simulink model "FCS_MPC_6ph_Regelungsmodell"  (R2022a)
settings: Solver=ode23t  StartTime=0.0  StopTime=0.1  RelTol=1e-3  AbsTol=1e-3  EnableMultiTasking=on
values from neighbouring files (symbols this model uses):
  f_c = 100000    [Params_testbench.m]
  L_d = 0.0001473    [Params_testbench.m]
  L_q = 0.0001484    [Params_testbench.m]
  L_x = 0.00005566    (= 5.566e-05)    [Params_testbench.m]
  L_y = L_x    (= 5.566e-05)    [Params_testbench.m]
  p = 5    [Params_testbench.m]
  psi_pm = 0.0048    [Params_testbench.m]
  R_ph = 0.1278    [Params_testbench.m]
  T_100MHz = 1/f_100MHz    (= 1e-08)    [Params_testbench.m]
  u_dc = 36.0    (= 36)    [Params_testbench.m]
libraries: hdlsllib x53, nesl_utility x39, fl_lib x32, ee_lib x12, simulink x8, spsAlphaBetaZerotodq0Lib x1
(part 4 of 8)

== system FCS_MPC_6ph_Regelungsmodell/Microcontroller Software/Phase_voltages_per_switching_state2 ==
  theta_el : Inport
  theta_el_offset_AXI : Inport  Port=2
  u_dc_link_voltage_AXI : Inport  Port=3
  Index : Inport  Port=4
  valid_in_delay_compensation : Inport  Port=5
  valid_in_min_cost_function-and_vopt : Inport  Port=6
  valid_in_ADC : Inport  Port=7
  Add4 : Sum  Inputs=+-  OutDataTypeStr=Inherit: Same as first input
  Add5 : Sum  Inputs=-+  OutDataTypeStr=Inherit: Same as first input
  Add6 : Sum  OutDataTypeStr=Inherit: Same as first input
  Compare Limit_High1 : simulink/Logic and Bit Operations/Compare To Constant  relop=>=  const=2*pi  OutDataTypeStr=boolean
  Compare Limit_Low1 : simulink/Logic and Bit Operations/Compare To Constant  relop=<  const=0  OutDataTypeStr=boolean
  Constant2 : Constant  Value=2*pi  OutDataTypeStr=single  SampleTime=1/100000000
  Constant3 : Constant  Value=2*pi  OutDataTypeStr=single  SampleTime=1/100000000
  Data Type Conversion34 : DataTypeConversion  OutDataTypeStr=single  SaturateOnIntegerOverflow=off  RndMeth=Floor
  Delay{1..11,13..14} (13 alike) : Delay  DelayLength=1
  Detect Rise Positive : hdlsllib/Logic and Bit Operations/Detect Rise Positive  vinit=0  OutDataTypeStr=boolean
      settings: SourceProductBaseCode=SL
  Detect Rise Positive1 : hdlsllib/Logic and Bit Operations/Detect Rise Positive  vinit=0  OutDataTypeStr=boolean
      settings: SourceProductBaseCode=SL
  Logical Operator : Logic  Operator=OR  AllPortsSameDT=off  OutDataTypeStr=boolean
  MATLAB Function1 : MATLAB Function  Commented=on  TreatAsAtomicUnit=on
  Mux{1..8} (8 alike) : Mux
  Mux16 : Mux  Inputs=8
  Sincos : Trigonometry  Operator=sincos
  Sine HDL Optimized : hdlsllib/Lookup Tables/Cosine HDL Optimized  Commented=on  OutputFormula=sin(2*pi*u) and cos(2*pi*u)  NumDataPoints=64  TableDataTypeStr=fixdt(1,24,20)  SimulateLUTROMDelay=off
      settings: SourceProductBaseCode=SL
  Subsystem : Subsystem
  Switch_Limit_High1 : Switch  Criteria=u2 > Threshold  SaturateOnIntegerOverflow=off  InputSameDT=off  OutDataTypeStr=Inherit: Same as first input
  Switch_Limit_Low1 : Switch  Criteria=u2 > Threshold  SaturateOnIntegerOverflow=off  InputSameDT=off  OutDataTypeStr=Inherit: Same as first input
  Switch_on1 : Switch  Threshold=1  OutDataTypeStr=single  RndMeth=Simplest  SaturateOnIntegerOverflow=off  InputSameDT=off
  Switch_on13 : Switch  Threshold=1  RndMeth=Simplest  SaturateOnIntegerOverflow=off  InputSameDT=off  OutDataTypeStr=Inherit: Same as first input
  Switch_on2 : Switch  Threshold=1  RndMeth=Simplest  SaturateOnIntegerOverflow=off  InputSameDT=off  OutDataTypeStr=Inherit: Same as first input
  Switch_on3 : Switch  Threshold=1  OutDataTypeStr=int32  RndMeth=Simplest  SaturateOnIntegerOverflow=off  InputSameDT=off
  done : Outport
  phase_voltages_per_switching_state : Outport  Port=2
  theta_test : Outport  Port=3
  wires:
  Delay14/1 -> Switch_on3/3
  Delay13/1 -> Switch_on13/3
  Switch_on13/1 -> Delay13/1, Add4/2
  u_dc_link_voltage_AXI/1 -> Delay8/1  "End_Cycle"
  Switch_on1/1 -> Subsystem/1(u_dc_link_voltage15), Delay1/1
  Detect Rise Positive1/1 -> Delay10/1, Switch_on3/2, Switch_on1/2  "End_Cycle"
  Delay1/1 -> Switch_on1/3
  Index/1 -> Delay9/1  "End_Cycle"
  Logical Operator/1 -> Detect Rise Positive1/1
  Switch_on3/1 -> Delay14/1, Subsystem/2(Index 15)
  Mux1/1 -> Mux16/1
  Mux2/1 -> Mux16/2
  Mux3/1 -> Mux16/3
  Mux4/1 -> Mux16/4
  Mux5/1 -> Mux16/5
  Mux6/1 -> Mux16/6
  Mux7/1 -> Mux16/7
  Mux8/1 -> Mux16/8
  Mux16/1 -> Delay11/1
  valid_in_ADC/1 -> Delay5/1
  valid_in_delay_compensation/1 -> Delay6/1
  valid_in_min_cost_function-and_vopt/1 -> Delay7/1
  theta_el/1 -> Delay3/1  "End_Cycle"
  Add4/1 -> Switch_Limit_High1/3, Add6/1, Compare Limit_Low1/1, Add5/2, Compare Limit_High1/1
  Compare Limit_Low1/1 -> Switch_Limit_Low1/2
  Add5/1 -> Switch_Limit_High1/1
  Switch_Limit_Low1/1 -> Data Type Conversion34/1  "End_Cycle"
  theta_el_offset_AXI/1 -> Delay4/1
  Constant3/1 -> Add6/2
  Constant2/1 -> Add5/1
  Compare Limit_High1/1 -> Switch_Limit_High1/2
  Add6/1 -> Switch_Limit_Low1/1
  Switch_Limit_High1/1 -> Switch_Limit_Low1/3
  Delay2/1 -> Switch_on2/3
  Switch_on2/1 -> Add4/1, Delay2/1
  Detect Rise Positive/1 -> Switch_on2/2, Switch_on13/2  "End_Cycle"
  Delay3/1 -> Switch_on2/1
  Delay4/1 -> Switch_on13/1
  Delay5/1 -> Detect Rise Positive/1
  Delay6/1 -> Logical Operator/1
  Delay7/1 -> Logical Operator/2
  Delay8/1 -> Switch_on1/1
  Delay9/1 -> Switch_on3/1
  Delay10/1 -> done/1
  Delay11/1 -> phase_voltages_per_switching_state/1
  Sincos/2 -> theta_test/1, Subsystem/4(cos_theta_el)
  Subsystem/1(d_voltage_per_switching_state) -> Mux1/1
  Subsystem/2(q_voltage_per_switching_state) -> Mux1/2
  Subsystem/3(x_voltage_per_switching_state) -> Mux1/3
  Subsystem/4(y_voltage_per_switching_state) -> Mux1/4
  Subsystem/5(d_voltage_per_switching_state1) -> Mux2/1
  Subsystem/6(q_voltage_per_switching_state1) -> Mux2/2
  Subsystem/7(x_voltage_per_switching_state1) -> Mux2/3
  Subsystem/8(y_voltage_per_switching_state1) -> Mux2/4
  Subsystem/9(d_voltage_per_switching_state2) -> Mux3/1
  Subsystem/10(q_voltage_per_switching_state2) -> Mux3/2
  Subsystem/11(x_voltage_per_switching_state2) -> Mux3/3
  Subsystem/12(y_voltage_per_switching_state2) -> Mux3/4
  Subsystem/13(d_voltage_per_switching_state3) -> Mux4/1
  Subsystem/14(q_voltage_per_switching_state3) -> Mux4/2
  Subsystem/15(x_voltage_per_switching_state3) -> Mux4/3
  Subsystem/16(y_voltage_per_switching_state3) -> Mux4/4
  Subsystem/17(d_voltage_per_switching_state4) -> Mux5/1
  Subsystem/18(q_voltage_per_switching_state4) -> Mux5/2
  Subsystem/19(x_voltage_per_switching_state4) -> Mux5/3
  Subsystem/20(y_voltage_per_switching_state4) -> Mux5/4
  Subsystem/21(d_voltage_per_switching_state5) -> Mux6/1
  Subsystem/22(q_voltage_per_switching_state5) -> Mux6/2
  Subsystem/23(x_voltage_per_switching_state5) -> Mux6/3
  Subsystem/24(y_voltage_per_switching_state5) -> Mux6/4
  Subsystem/25(d_voltage_per_switching_state6) -> Mux7/1
  Subsystem/26(q_voltage_per_switching_state6) -> Mux7/2
  Subsystem/27(x_voltage_per_switching_state6) -> Mux7/3
  Subsystem/28(y_voltage_per_switching_state6) -> Mux7/4
  Subsystem/29(d_voltage_per_switching_state7) -> Mux8/1
  Subsystem/30(q_voltage_per_switching_state7) -> Mux8/2
  Subsystem/31(x_voltage_per_switching_state7) -> Mux8/3
  Subsystem/32(y_voltage_per_switching_state7) -> Mux8/4
  Sincos/1 -> Subsystem/3(sin_theta_el)
  Data Type Conversion34/1 -> Sincos/1

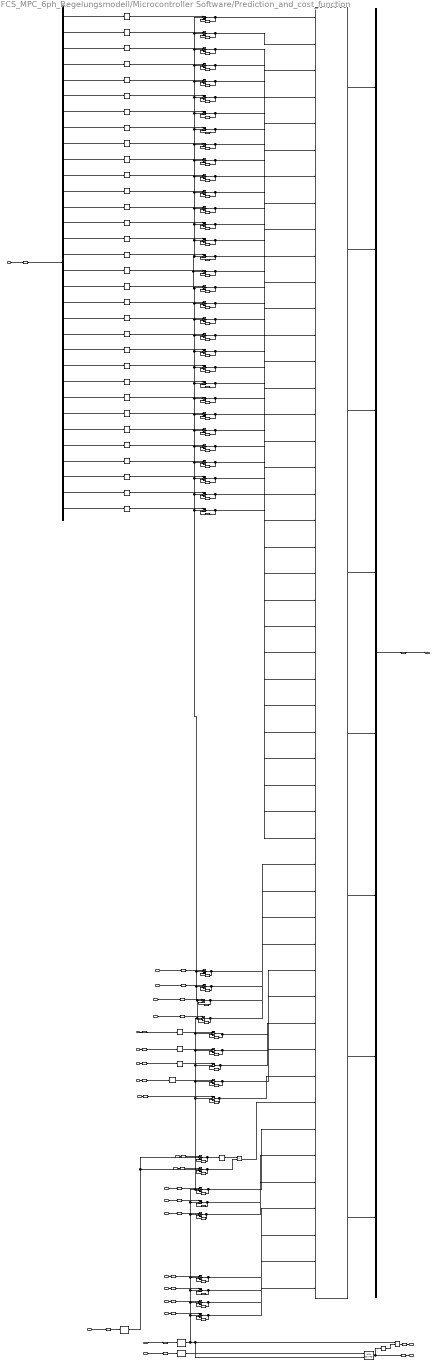
== system FCS_MPC_6ph_Regelungsmodell/Microcontroller Software/Prediction_and_cost_function ==
  Lq_AXI : Inport
  Ld_AXI : Inport  Port=2
  SampleTime_div_Ld_AXI : Inport  Port=3
  SampleTime_div_Lq_AXI : Inport  Port=4
  SampleTime_div_Lx_AXI : Inport  Port=5
  SampleTime_div_Ly_AXI : Inport  Port=6
  id_k_1 : Inport  Port=7
  iq_k_1 : Inport  Port=8
  ix_k_1 : Inport  Port=9
  iy_k_1 : Inport  Port=10
  Rs_AXI : Inport  Port=11
  omega_m_measured : Inport  Port=12
  pole_pairs_AXI : Inport  Port=13
  psiPM_AXI : Inport  Port=14
  id_ref_AXI : Inport  Port=15
  iq_ref_AXI : Inport  Port=16
  ix_ref_AXI : Inport  Port=17
  iy_ref_AXI : Inport  Port=18
  valid_in : Inport  Port=19
  Reset : Inport  Port=20
  valid_in_ADC : Inport  Port=21
  dqxy_phase_voltage_per_switching_state : Inport  Port=22
  Compare To Constant : hdlsllib/Logic and Bit Operations/Compare To Constant  relop=<=  const=8  OutDataTypeStr=boolean
      settings: SourceProductBaseCode=SL
  Data Type Conversion{1..17,19..38} (37 alike) : DataTypeConversion  OutDataTypeStr=single  RndMeth=Nearest  SaturateOnIntegerOverflow=off
  Delay{1..4,8..37,42..45,51,57,59..60,68,104..135} (75 alike) : Delay  DelayLength=1
  Demux : Demux  Outputs=32
  Detect Rise Positive : hdlsllib/Logic and Bit Operations/Detect Rise Positive  vinit=0  OutDataTypeStr=boolean
      settings: SourceProductBaseCode=SL
  Detect Rise Positive1 : hdlsllib/Logic and Bit Operations/Detect Rise Positive  vinit=0  OutDataTypeStr=boolean
      settings: SourceProductBaseCode=SL
  Detect Rise Positive2 : hdlsllib/Logic and Bit Operations/Detect Rise Positive  vinit=0  OutDataTypeStr=boolean
      settings: SourceProductBaseCode=SL
  HDL Counter : hdlsllib/Sources/HDL Counter  CountType=Free running  CountInit=0  CountStep=1  CountMax=25  CountFromType=Initial value  CountFrom=0  CountResetPort=on  CountLoadPort=off  CountEnbPort=on  CountDirPort=off  CountHitOutputPort=off  CountDataType=Signed  CountWordLen=32  CountFracLen=0  CountSampTime=1
  Logical Operator : Logic  AllPortsSameDT=off  OutDataTypeStr=boolean
  Mux : Mux  Inputs=8
  Product : Product  Inputs=**
  Subsystem : Subsystem
  Switch_on{1..4,8..10,12..21,59..90} (49 alike) : Switch  Threshold=1  OutDataTypeStr=single  RndMeth=Simplest  SaturateOnIntegerOverflow=off  InputSameDT=off
  Switch_on11 : Switch  Threshold=1  RndMeth=Simplest  SaturateOnIntegerOverflow=off  InputSameDT=off  OutDataTypeStr=Inherit: Same as first input
  done : Outport
  Index : Outport  Port=2
  J : Outport  Port=3
  wires:
  Switch_on12/1 -> Subsystem/41(Rs15), Delay12/1
  Rs_AXI/1 -> Delay31/1
  Delay31/1 -> Switch_on12/1
  Delay23/1 -> Switch_on21/1
  Delay3/1 -> Switch_on3/3
  Delay10/1 -> Switch_on10/3
  Delay43/1 -> Switch_on2/1
  Delay17/1 -> Switch_on18/3
  Switch_on10/1 -> Delay10/1, Subsystem/43(Lq15)
  Delay11/1 -> Switch_on11/3
  Delay24/1 -> Switch_on20/1
  Delay36/1 -> Switch_on9/1
  Delay37/1 -> Switch_on8/1
  Delay1/1 -> Switch_on1/3
  Delay42/1 -> Switch_on3/1
  Product/1 -> Subsystem/42(omega_el15)  "omega_el"
  valid_in/1 -> Delay21/1
  Delay9/1 -> Switch_on9/3
  iy_k_1/1 -> Delay30/1
  Delay20/1 -> Switch_on21/3
  Delay35/1 -> Switch_on4/1
  pole_pairs_AXI/1 -> Delay35/1
  omega_m_measured/1 -> Delay51/1
  Switch_on18/1 -> Delay17/1, Subsystem/36(SampleTime_div_Ly15)
  Delay19/1 -> Switch_on20/3
  Delay13/1 -> Switch_on13/3
  Switch_on15/1 -> Delay14/1, Subsystem/39(ix_k_16)
  Delay18/1 -> Switch_on19/3
  Lq_AXI/1 -> Delay34/1
  Switch_on19/1 -> Delay18/1, Subsystem/35(SampleTime_div_Lx15)
  Switch_on20/1 -> Delay19/1, Subsystem/34(SampleTime_div_Lq15)
  Switch_on13/1 -> Delay13/1, Subsystem/40(iy_k_16)
  ix_k_1/1 -> Delay29/1
  Delay45/1 -> Switch_on14/1
  Delay2/1 -> Switch_on2/3
  Delay16/1 -> Switch_on17/3
  Switch_on17/1 -> Delay16/1, Subsystem/37(id_k_16)
  iq_k_1/1 -> Delay28/1
  Delay15/1 -> Switch_on16/3
  Switch_on16/1 -> Delay15/1, Subsystem/38(iq_k_16)
  iq_ref_AXI/1 -> Delay43/1
  Switch_on11/1 -> Data Type Conversion4/1, Delay11/1
  Delay33/1 -> Switch_on14/3
  Ld_AXI/1 -> Delay36/1
  Delay25/1 -> Switch_on19/1
  psiPM_AXI/1 -> Delay37/1
  Switch_on14/1 -> Delay33/1, Subsystem/49(iy_ref15)
  Delay12/1 -> Switch_on12/3
  Delay21/1 -> Detect Rise Positive/1
  Switch_on3/1 -> Delay3/1, Subsystem/46(id_ref15)
  Switch_on21/1 -> Delay20/1, Subsystem/33(SampleTime_div_Ld15)
  Switch_on2/1 -> Delay2/1, Subsystem/47(iq_ref15)
  Delay34/1 -> Switch_on10/1
  iy_ref_AXI/1 -> Delay45/1
  Switch_on1/1 -> Delay1/1, Subsystem/48(ix_ref15)
  id_k_1/1 -> Delay27/1
  ix_ref_AXI/1 -> Delay44/1
  Switch_on9/1 -> Delay9/1, Subsystem/44(Ld15)
  Delay26/1 -> Switch_on18/1
  Delay14/1 -> Switch_on15/3
  id_ref_AXI/1 -> Delay42/1
  Delay44/1 -> Switch_on1/1
  Switch_on8/1 -> Delay8/1, Subsystem/45(psiPM15)
  Delay8/1 -> Switch_on8/3
  Delay27/1 -> Data Type Conversion7/1
  Delay28/1 -> Data Type Conversion8/1
  Delay29/1 -> Data Type Conversion9/1
  Delay30/1 -> Data Type Conversion10/1
  Delay51/1 -> Switch_on11/1
  SampleTime_div_Ld_AXI/1 -> Delay23/1
  SampleTime_div_Lq_AXI/1 -> Delay24/1
  SampleTime_div_Lx_AXI/1 -> Delay25/1
  SampleTime_div_Ly_AXI/1 -> Delay26/1
  Reset/1 -> Delay57/1
  Delay57/1 -> Detect Rise Positive1/1
  Detect Rise Positive1/1 -> HDL Counter/1  "End_Cycle"
  HDL Counter/1 -> Compare To Constant/1, Delay59/1
  Compare To Constant/1 -> Logical Operator/2
  Logical Operator/1 -> Delay22/1
  Delay59/1 -> Index/1
  valid_in_ADC/1 -> Delay60/1
  Delay60/1 -> Detect Rise Positive2/1
  Mux/1 -> Delay68/1
  Delay68/1 -> J/1
  Switch_on61/1 -> Subsystem/30(q_phase_voltage_per_switching_state7), Delay106/1
  Delay106/1 -> Switch_on61/3
  Delay107/1 -> Switch_on62/3
  Switch_on62/1 -> Subsystem/29(d_phase_voltage_per_switching_state7), Delay107/1
  Delay104/1 -> Switch_on59/3
  Switch_on59/1 -> Subsystem/32(y_phase_voltage_per_switching_state7), Delay104/1
  Delay105/1 -> Switch_on60/3
  Switch_on60/1 -> Subsystem/31(x_phase_voltage_per_switching_state7), Delay105/1
  Switch_on65/1 -> Subsystem/26(q_phase_voltage_per_switching_state6), Delay110/1
  Delay110/1 -> Switch_on65/3
  Delay111/1 -> Switch_on66/3
  Switch_on66/1 -> Subsystem/25(d_phase_voltage_per_switching_state6), Delay111/1
  Delay108/1 -> Switch_on63/3
  Switch_on63/1 -> Subsystem/28(y_phase_voltage_per_switching_state6), Delay108/1
  Delay109/1 -> Switch_on64/3
  Switch_on64/1 -> Subsystem/27(x_phase_voltage_per_switching_state6), Delay109/1
  Switch_on69/1 -> Subsystem/22(q_phase_voltage_per_switching_state5), Delay114/1
  Delay114/1 -> Switch_on69/3
  Delay115/1 -> Switch_on70/3
  Switch_on70/1 -> Subsystem/21(d_phase_voltage_per_switching_state5), Delay115/1
  Delay112/1 -> Switch_on67/3
  Switch_on67/1 -> Subsystem/24(y_phase_voltage_per_switching_state5), Delay112/1
  Delay113/1 -> Switch_on68/3
  Switch_on68/1 -> Subsystem/23(x_phase_voltage_per_switching_state5), Delay113/1
  Switch_on73/1 -> Subsystem/18(q_phase_voltage_per_switching_state4), Delay118/1
  Delay118/1 -> Switch_on73/3
  Delay119/1 -> Switch_on74/3
  Switch_on74/1 -> Subsystem/17(d_phase_voltage_per_switching_state4), Delay119/1
  Delay116/1 -> Switch_on71/3
  Switch_on71/1 -> Subsystem/20(y_phase_voltage_per_switching_state4), Delay116/1
  Delay117/1 -> Switch_on72/3
  Switch_on72/1 -> Subsystem/19(x_phase_voltage_per_switching_state4), Delay117/1
  Switch_on77/1 -> Subsystem/14(q_phase_voltage_per_switching_state3), Delay122/1
  Delay122/1 -> Switch_on77/3
  Delay123/1 -> Switch_on78/3
  Switch_on78/1 -> Subsystem/13(d_phase_voltage_per_switching_state3), Delay123/1
  Delay120/1 -> Switch_on75/3
  Switch_on75/1 -> Subsystem/16(y_phase_voltage_per_switching_state3), Delay120/1
  Delay121/1 -> Switch_on76/3
  Switch_on76/1 -> Subsystem/15(x_phase_voltage_per_switching_state3), Delay121/1
  Switch_on81/1 -> Subsystem/10(q_phase_voltage_per_switching_state2), Delay126/1
  Delay126/1 -> Switch_on81/3
  Delay127/1 -> Switch_on82/3
  Switch_on82/1 -> Subsystem/9(d_phase_voltage_per_switching_state2), Delay127/1
  Delay124/1 -> Switch_on79/3
  Switch_on79/1 -> Subsystem/12(y_phase_voltage_per_switching_state2), Delay124/1
  Delay125/1 -> Switch_on80/3
  Switch_on80/1 -> Subsystem/11(x_phase_voltage_per_switching_state2), Delay125/1
  Switch_on85/1 -> Subsystem/6(q_phase_voltage_per_switching_state1), Delay130/1
  Delay130/1 -> Switch_on85/3
  Delay131/1 -> Switch_on86/3
  Switch_on86/1 -> Subsystem/5(d_phase_voltage_per_switching_state1), Delay131/1
  Delay128/1 -> Switch_on83/3
  Switch_on83/1 -> Subsystem/8(y_phase_voltage_per_switching_state1), Delay128/1
  Delay129/1 -> Switch_on84/3
  Switch_on84/1 -> Subsystem/7(x_phase_voltage_per_switching_state1), Delay129/1
  Switch_on89/1 -> Subsystem/2(q_phase_voltage_per_switching_state), Delay134/1
  Delay134/1 -> Switch_on89/3
  Delay135/1 -> Switch_on90/3
  Switch_on90/1 -> Subsystem/1(d_phase_voltage_per_switching_state), Delay135/1
  Delay132/1 -> Switch_on87/3
  Switch_on87/1 -> Subsystem/4(y_phase_voltage_per_switching_state), Delay132/1
  Delay133/1 -> Switch_on88/3
  Switch_on88/1 -> Subsystem/3(x_phase_voltage_per_switching_state), Delay133/1
  Detect Rise Positive/1 -> Logical Operator/1, HDL Counter/2, Switch_on14/2, Switch_on1/2, Switch_on8/2, Switch_on9/2, Switch_on12/2, Switch_on20/2, Switch_on90/2, Switch_on89/2, Switch_on88/2, Switch_on87/2, Switch_on86/2, Switch_on85/2, Switch_on84/2, Switch_on83/2, Switch_on82/2, Switch_on81/2, Switch_on80/2, Switch_on79/2, Switch_on78/2, Switch_on77/2, Switch_on76/2, Switch_on75/2, Switch_on74/2, Switch_on73/2, Switch_on72/2, Switch_on71/2, Switch_on70/2, Switch_on69/2, Switch_on68/2, Switch_on67/2, Switch_on66/2, Switch_on65/2, Switch_on64/2, Switch_on63/2, Switch_on62/2, Switch_on61/2, Switch_on60/2, Switch_on59/2, Switch_on21/2, Switch_on19/2, Switch_on18/2, Switch_on17/2, Switch_on16/2, Switch_on15/2, Switch_on13/2, Switch_on10/2, Switch_on3/2, Switch_on2/2  "End_Cycle"
  Demux/32 -> Data Type Conversion38/1
  Demux/31 -> Data Type Conversion37/1
  Demux/30 -> Data Type Conversion36/1
  Demux/29 -> Data Type Conversion35/1
  Demux/28 -> Data Type Conversion34/1
  Demux/27 -> Data Type Conversion33/1
  Demux/26 -> Data Type Conversion32/1
  Demux/25 -> Data Type Conversion31/1
  Demux/24 -> Data Type Conversion30/1
  Demux/23 -> Data Type Conversion29/1
  Demux/22 -> Data Type Conversion28/1
  Demux/21 -> Data Type Conversion27/1
  Demux/20 -> Data Type Conversion26/1
  Demux/19 -> Data Type Conversion25/1
  Demux/18 -> Data Type Conversion24/1
  Demux/17 -> Data Type Conversion23/1
  Demux/16 -> Data Type Conversion22/1
  Demux/15 -> Data Type Conversion21/1
  Demux/14 -> Data Type Conversion20/1
  Demux/13 -> Data Type Conversion19/1
  Demux/12 -> Data Type Conversion17/1
  Demux/11 -> Data Type Conversion16/1
  Demux/10 -> Data Type Conversion15/1
  Demux/9 -> Data Type Conversion14/1
  Demux/8 -> Data Type Conversion13/1
  Demux/7 -> Data Type Conversion12/1
  Demux/6 -> Data Type Conversion11/1
  Demux/5 -> Data Type Conversion6/1
  Demux/4 -> Data Type Conversion5/1
  Demux/3 -> Data Type Conversion3/1
  Demux/2 -> Data Type Conversion2/1
  Demux/1 -> Data Type Conversion1/1
  dqxy_phase_voltage_per_switching_state/1 -> Delay32/1
  Delay22/1 -> done/1
  Delay32/1 -> Demux/1
  Data Type Conversion10/1 -> Switch_on13/1
  Data Type Conversion9/1 -> Switch_on15/1
  Data Type Conversion8/1 -> Switch_on16/1
  Data Type Conversion7/1 -> Switch_on17/1
  Data Type Conversion4/1 -> Product/1
  Data Type Conversion38/1 -> Switch_on59/1
  Data Type Conversion37/1 -> Switch_on60/1
  Data Type Conversion36/1 -> Switch_on61/1
  Data Type Conversion35/1 -> Switch_on62/1
  Data Type Conversion34/1 -> Switch_on63/1
  Data Type Conversion33/1 -> Switch_on64/1
  Data Type Conversion32/1 -> Switch_on65/1
  Data Type Conversion31/1 -> Switch_on66/1
  Data Type Conversion30/1 -> Switch_on67/1
  Data Type Conversion29/1 -> Switch_on68/1
  Data Type Conversion28/1 -> Switch_on69/1
  Data Type Conversion27/1 -> Switch_on70/1
  Data Type Conversion26/1 -> Switch_on71/1
  Data Type Conversion25/1 -> Switch_on72/1
  Data Type Conversion24/1 -> Switch_on73/1
  Data Type Conversion23/1 -> Switch_on74/1
  Data Type Conversion22/1 -> Switch_on75/1
  Data Type Conversion21/1 -> Switch_on76/1
  Data Type Conversion20/1 -> Switch_on77/1
  Data Type Conversion19/1 -> Switch_on78/1
  Data Type Conversion17/1 -> Switch_on79/1
  Data Type Conversion16/1 -> Switch_on80/1
  Data Type Conversion15/1 -> Switch_on81/1
  Data Type Conversion14/1 -> Switch_on82/1
  Data Type Conversion13/1 -> Switch_on83/1
  Data Type Conversion12/1 -> Switch_on84/1
  Data Type Conversion11/1 -> Switch_on85/1
  Data Type Conversion6/1 -> Switch_on86/1
  Data Type Conversion5/1 -> Switch_on87/1
  Data Type Conversion3/1 -> Switch_on88/1
  Data Type Conversion2/1 -> Switch_on89/1
  Data Type Conversion1/1 -> Switch_on90/1
  Subsystem/8(J7) -> Mux/8
  Subsystem/7(J6) -> Mux/7
  Subsystem/6(J5) -> Mux/6
  Subsystem/5(J4) -> Mux/5
  Subsystem/4(J3) -> Mux/4
  Subsystem/3(J2) -> Mux/3
  Subsystem/2(J1) -> Mux/2
  Subsystem/1(J) -> Mux/1
  Detect Rise Positive2/1 -> Switch_on4/2, Switch_on11/2  "End_Cycle"
  Switch_on4/1 -> Product/2, Delay4/1
  Delay4/1 -> Switch_on4/3

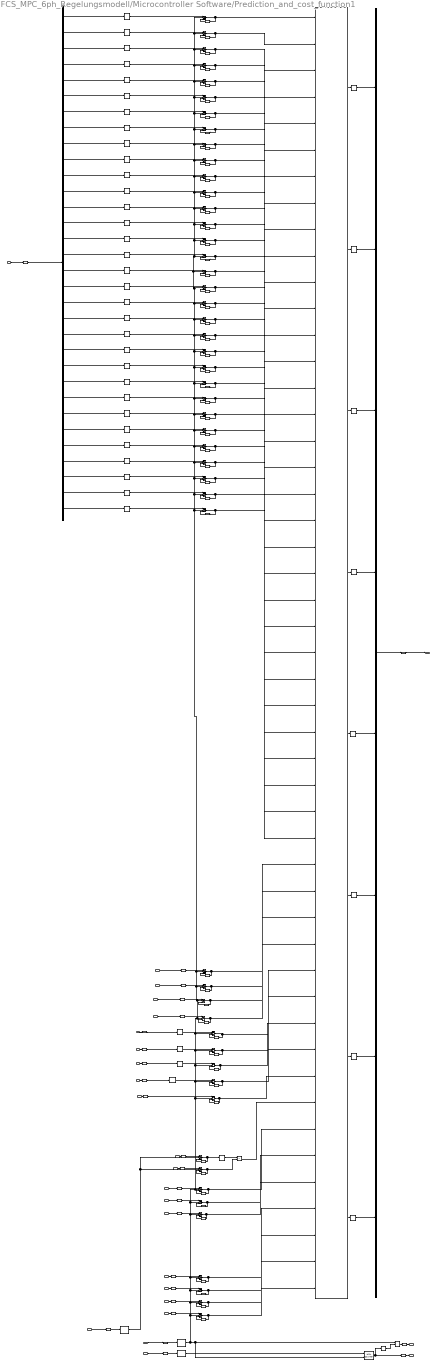
== system FCS_MPC_6ph_Regelungsmodell/Microcontroller Software/Prediction_and_cost_function1 ==
  Lq_AXI : Inport
  Ld_AXI : Inport  Port=2
  SampleTime_div_Ld_AXI : Inport  Port=3
  SampleTime_div_Lq_AXI : Inport  Port=4
  SampleTime_div_Lx_AXI : Inport  Port=5
  SampleTime_div_Ly_AXI : Inport  Port=6
  id_k_1 : Inport  Port=7
  iq_k_1 : Inport  Port=8
  ix_k_1 : Inport  Port=9
  iy_k_1 : Inport  Port=10
  Rs_AXI : Inport  Port=11
  omega_m_measured : Inport  Port=12
  pole_pairs_AXI : Inport  Port=13
  psiPM_AXI : Inport  Port=14
  id_ref_AXI : Inport  Port=15
  iq_ref_AXI : Inport  Port=16
  ix_ref_AXI : Inport  Port=17
  iy_ref_AXI : Inport  Port=18
  valid_in : Inport  Port=19
  Reset : Inport  Port=20
  valid_in_ADC : Inport  Port=21
  dqxy_phase_voltage_per_switching_state : Inport  Port=22
  Compare To Constant : hdlsllib/Logic and Bit Operations/Compare To Constant  relop=<=  const=8  OutDataTypeStr=boolean
      settings: SourceProductBaseCode=SL
  Data Type Conversion{1..17,19..38} (37 alike) : DataTypeConversion  OutDataTypeStr=single  RndMeth=Nearest  SaturateOnIntegerOverflow=off
  Data Type Conversion{39..46} (8 alike) : DataTypeConversion  OutDataTypeStr=fixdt(1,20,11)  RndMeth=Nearest  SaturateOnIntegerOverflow=off
  Delay{1..4,8..37,42..45,51,57,59..60,68,104..135} (75 alike) : Delay  DelayLength=1
  Demux : Demux  Outputs=32
  Detect Rise Positive : hdlsllib/Logic and Bit Operations/Detect Rise Positive  vinit=0  OutDataTypeStr=boolean
      settings: SourceProductBaseCode=SL
  Detect Rise Positive1 : hdlsllib/Logic and Bit Operations/Detect Rise Positive  vinit=0  OutDataTypeStr=boolean
      settings: SourceProductBaseCode=SL
  Detect Rise Positive2 : hdlsllib/Logic and Bit Operations/Detect Rise Positive  vinit=0  OutDataTypeStr=boolean
      settings: SourceProductBaseCode=SL
  HDL Counter : hdlsllib/Sources/HDL Counter  CountType=Free running  CountInit=0  CountStep=1  CountMax=25  CountFromType=Initial value  CountFrom=0  CountResetPort=on  CountLoadPort=off  CountEnbPort=on  CountDirPort=off  CountHitOutputPort=off  CountDataType=Signed  CountWordLen=32  CountFracLen=0  CountSampTime=1
  Logical Operator : Logic  AllPortsSameDT=off  OutDataTypeStr=boolean
  Mux : Mux  Inputs=8
  Product : Product  Inputs=**
  Subsystem : Subsystem
  Switch_on{1..4,8..10,12..21,59..90} (49 alike) : Switch  Threshold=1  OutDataTypeStr=single  RndMeth=Simplest  SaturateOnIntegerOverflow=off  InputSameDT=off
  Switch_on11 : Switch  Threshold=1  RndMeth=Simplest  SaturateOnIntegerOverflow=off  InputSameDT=off  OutDataTypeStr=Inherit: Same as first input
  done : Outport
  Index : Outport  Port=2
  J : Outport  Port=3
  wires:
  Switch_on12/1 -> Subsystem/41(Rs15), Delay12/1
  Rs_AXI/1 -> Delay31/1
  Delay31/1 -> Switch_on12/1
  Delay23/1 -> Switch_on21/1
  Delay3/1 -> Switch_on3/3
  Delay10/1 -> Switch_on10/3
  Delay43/1 -> Switch_on2/1
  Delay17/1 -> Switch_on18/3
  Switch_on10/1 -> Delay10/1, Subsystem/43(Lq15)
  Delay11/1 -> Switch_on11/3
  Delay24/1 -> Switch_on20/1
  Delay36/1 -> Switch_on9/1
  Delay37/1 -> Switch_on8/1
  Delay1/1 -> Switch_on1/3
  Delay42/1 -> Switch_on3/1
  Product/1 -> Subsystem/42(omega_el15)  "omega_el"
  valid_in/1 -> Delay21/1
  Delay9/1 -> Switch_on9/3
  iy_k_1/1 -> Delay30/1
  Delay20/1 -> Switch_on21/3
  Delay35/1 -> Switch_on4/1
  pole_pairs_AXI/1 -> Delay35/1
  omega_m_measured/1 -> Delay51/1
  Switch_on18/1 -> Delay17/1, Subsystem/36(SampleTime_div_Ly15)
  Delay19/1 -> Switch_on20/3
  Delay13/1 -> Switch_on13/3
  Switch_on15/1 -> Delay14/1, Subsystem/39(ix_k_16)
  Delay18/1 -> Switch_on19/3
  Lq_AXI/1 -> Delay34/1
  Switch_on19/1 -> Delay18/1, Subsystem/35(SampleTime_div_Lx15)
  Switch_on20/1 -> Delay19/1, Subsystem/34(SampleTime_div_Lq15)
  Switch_on13/1 -> Delay13/1, Subsystem/40(iy_k_16)
  ix_k_1/1 -> Delay29/1
  Delay45/1 -> Switch_on14/1
  Delay2/1 -> Switch_on2/3
  Delay16/1 -> Switch_on17/3
  Switch_on17/1 -> Delay16/1, Subsystem/37(id_k_16)
  iq_k_1/1 -> Delay28/1
  Delay15/1 -> Switch_on16/3
  Switch_on16/1 -> Delay15/1, Subsystem/38(iq_k_16)
  iq_ref_AXI/1 -> Delay43/1
  Switch_on11/1 -> Data Type Conversion4/1, Delay11/1
  Delay33/1 -> Switch_on14/3
  Ld_AXI/1 -> Delay36/1
  Delay25/1 -> Switch_on19/1
  psiPM_AXI/1 -> Delay37/1
  Switch_on14/1 -> Delay33/1, Subsystem/49(iy_ref15)
  Delay12/1 -> Switch_on12/3
  Delay21/1 -> Detect Rise Positive/1
  Switch_on3/1 -> Delay3/1, Subsystem/46(id_ref15)
  Switch_on21/1 -> Delay20/1, Subsystem/33(SampleTime_div_Ld15)
  Switch_on2/1 -> Delay2/1, Subsystem/47(iq_ref15)
  Delay34/1 -> Switch_on10/1
  iy_ref_AXI/1 -> Delay45/1
  Switch_on1/1 -> Delay1/1, Subsystem/48(ix_ref15)
  id_k_1/1 -> Delay27/1
  ix_ref_AXI/1 -> Delay44/1
  Switch_on9/1 -> Delay9/1, Subsystem/44(Ld15)
  Delay26/1 -> Switch_on18/1
  Delay14/1 -> Switch_on15/3
  id_ref_AXI/1 -> Delay42/1
  Delay44/1 -> Switch_on1/1
  Switch_on8/1 -> Delay8/1, Subsystem/45(psiPM15)
  Delay8/1 -> Switch_on8/3
  Delay27/1 -> Data Type Conversion7/1
  Delay28/1 -> Data Type Conversion8/1
  Delay29/1 -> Data Type Conversion9/1
  Delay30/1 -> Data Type Conversion10/1
  Delay51/1 -> Switch_on11/1
  SampleTime_div_Ld_AXI/1 -> Delay23/1
  SampleTime_div_Lq_AXI/1 -> Delay24/1
  SampleTime_div_Lx_AXI/1 -> Delay25/1
  SampleTime_div_Ly_AXI/1 -> Delay26/1
  Reset/1 -> Delay57/1
  Delay57/1 -> Detect Rise Positive1/1
  Detect Rise Positive1/1 -> HDL Counter/1  "End_Cycle"
  HDL Counter/1 -> Compare To Constant/1, Delay59/1
  Compare To Constant/1 -> Logical Operator/2
  Logical Operator/1 -> Delay22/1
  Delay59/1 -> Index/1
  valid_in_ADC/1 -> Delay60/1
  Delay60/1 -> Detect Rise Positive2/1
  Mux/1 -> Delay68/1
  Delay68/1 -> J/1
  Switch_on61/1 -> Subsystem/30(q_phase_voltage_per_switching_state7), Delay106/1
  Delay106/1 -> Switch_on61/3
  Delay107/1 -> Switch_on62/3
  Switch_on62/1 -> Subsystem/29(d_phase_voltage_per_switching_state7), Delay107/1
  Delay104/1 -> Switch_on59/3
  Switch_on59/1 -> Subsystem/32(y_phase_voltage_per_switching_state7), Delay104/1
  Delay105/1 -> Switch_on60/3
  Switch_on60/1 -> Subsystem/31(x_phase_voltage_per_switching_state7), Delay105/1
  Switch_on65/1 -> Subsystem/26(q_phase_voltage_per_switching_state6), Delay110/1
  Delay110/1 -> Switch_on65/3
  Delay111/1 -> Switch_on66/3
  Switch_on66/1 -> Subsystem/25(d_phase_voltage_per_switching_state6), Delay111/1
  Delay108/1 -> Switch_on63/3
  Switch_on63/1 -> Subsystem/28(y_phase_voltage_per_switching_state6), Delay108/1
  Delay109/1 -> Switch_on64/3
  Switch_on64/1 -> Subsystem/27(x_phase_voltage_per_switching_state6), Delay109/1
  Switch_on69/1 -> Subsystem/22(q_phase_voltage_per_switching_state5), Delay114/1
  Delay114/1 -> Switch_on69/3
  Delay115/1 -> Switch_on70/3
  Switch_on70/1 -> Subsystem/21(d_phase_voltage_per_switching_state5), Delay115/1
  Delay112/1 -> Switch_on67/3
  Switch_on67/1 -> Subsystem/24(y_phase_voltage_per_switching_state5), Delay112/1
  Delay113/1 -> Switch_on68/3
  Switch_on68/1 -> Subsystem/23(x_phase_voltage_per_switching_state5), Delay113/1
  Switch_on73/1 -> Subsystem/18(q_phase_voltage_per_switching_state4), Delay118/1
  Delay118/1 -> Switch_on73/3
  Delay119/1 -> Switch_on74/3
  Switch_on74/1 -> Subsystem/17(d_phase_voltage_per_switching_state4), Delay119/1
  Delay116/1 -> Switch_on71/3
  Switch_on71/1 -> Subsystem/20(y_phase_voltage_per_switching_state4), Delay116/1
  Delay117/1 -> Switch_on72/3
  Switch_on72/1 -> Subsystem/19(x_phase_voltage_per_switching_state4), Delay117/1
  Switch_on77/1 -> Subsystem/14(q_phase_voltage_per_switching_state3), Delay122/1
  Delay122/1 -> Switch_on77/3
  Delay123/1 -> Switch_on78/3
  Switch_on78/1 -> Subsystem/13(d_phase_voltage_per_switching_state3), Delay123/1
  Delay120/1 -> Switch_on75/3
  Switch_on75/1 -> Subsystem/16(y_phase_voltage_per_switching_state3), Delay120/1
  Delay121/1 -> Switch_on76/3
  Switch_on76/1 -> Subsystem/15(x_phase_voltage_per_switching_state3), Delay121/1
  Switch_on81/1 -> Subsystem/10(q_phase_voltage_per_switching_state2), Delay126/1
  Delay126/1 -> Switch_on81/3
  Delay127/1 -> Switch_on82/3
  Switch_on82/1 -> Subsystem/9(d_phase_voltage_per_switching_state2), Delay127/1
  Delay124/1 -> Switch_on79/3
  Switch_on79/1 -> Subsystem/12(y_phase_voltage_per_switching_state2), Delay124/1
  Delay125/1 -> Switch_on80/3
  Switch_on80/1 -> Subsystem/11(x_phase_voltage_per_switching_state2), Delay125/1
  Switch_on85/1 -> Subsystem/6(q_phase_voltage_per_switching_state1), Delay130/1
  Delay130/1 -> Switch_on85/3
  Delay131/1 -> Switch_on86/3
  Switch_on86/1 -> Subsystem/5(d_phase_voltage_per_switching_state1), Delay131/1
  Delay128/1 -> Switch_on83/3
  Switch_on83/1 -> Subsystem/8(y_phase_voltage_per_switching_state1), Delay128/1
  Delay129/1 -> Switch_on84/3
  Switch_on84/1 -> Subsystem/7(x_phase_voltage_per_switching_state1), Delay129/1
  Switch_on89/1 -> Subsystem/2(q_phase_voltage_per_switching_state), Delay134/1
  Delay134/1 -> Switch_on89/3
  Delay135/1 -> Switch_on90/3
  Switch_on90/1 -> Subsystem/1(d_phase_voltage_per_switching_state), Delay135/1
  Delay132/1 -> Switch_on87/3
  Switch_on87/1 -> Subsystem/4(y_phase_voltage_per_switching_state), Delay132/1
  Delay133/1 -> Switch_on88/3
  Switch_on88/1 -> Subsystem/3(x_phase_voltage_per_switching_state), Delay133/1
  Detect Rise Positive/1 -> Logical Operator/1, HDL Counter/2, Switch_on14/2, Switch_on1/2, Switch_on8/2, Switch_on9/2, Switch_on12/2, Switch_on20/2, Switch_on90/2, Switch_on89/2, Switch_on88/2, Switch_on87/2, Switch_on86/2, Switch_on85/2, Switch_on84/2, Switch_on83/2, Switch_on82/2, Switch_on81/2, Switch_on80/2, Switch_on79/2, Switch_on78/2, Switch_on77/2, Switch_on76/2, Switch_on75/2, Switch_on74/2, Switch_on73/2, Switch_on72/2, Switch_on71/2, Switch_on70/2, Switch_on69/2, Switch_on68/2, Switch_on67/2, Switch_on66/2, Switch_on65/2, Switch_on64/2, Switch_on63/2, Switch_on62/2, Switch_on61/2, Switch_on60/2, Switch_on59/2, Switch_on21/2, Switch_on19/2, Switch_on18/2, Switch_on17/2, Switch_on16/2, Switch_on15/2, Switch_on13/2, Switch_on10/2, Switch_on3/2, Switch_on2/2  "End_Cycle"
  Demux/32 -> Data Type Conversion38/1
  Demux/31 -> Data Type Conversion37/1
  Demux/30 -> Data Type Conversion36/1
  Demux/29 -> Data Type Conversion35/1
  Demux/28 -> Data Type Conversion34/1
  Demux/27 -> Data Type Conversion33/1
  Demux/26 -> Data Type Conversion32/1
  Demux/25 -> Data Type Conversion31/1
  Demux/24 -> Data Type Conversion30/1
  Demux/23 -> Data Type Conversion29/1
  Demux/22 -> Data Type Conversion28/1
  Demux/21 -> Data Type Conversion27/1
  Demux/20 -> Data Type Conversion26/1
  Demux/19 -> Data Type Conversion25/1
  Demux/18 -> Data Type Conversion24/1
  Demux/17 -> Data Type Conversion23/1
  Demux/16 -> Data Type Conversion22/1
  Demux/15 -> Data Type Conversion21/1
  Demux/14 -> Data Type Conversion20/1
  Demux/13 -> Data Type Conversion19/1
  Demux/12 -> Data Type Conversion17/1
  Demux/11 -> Data Type Conversion16/1
  Demux/10 -> Data Type Conversion15/1
  Demux/9 -> Data Type Conversion14/1
  Demux/8 -> Data Type Conversion13/1
  Demux/7 -> Data Type Conversion12/1
  Demux/6 -> Data Type Conversion11/1
  Demux/5 -> Data Type Conversion6/1
  Demux/4 -> Data Type Conversion5/1
  Demux/3 -> Data Type Conversion3/1
  Demux/2 -> Data Type Conversion2/1
  Demux/1 -> Data Type Conversion1/1
  dqxy_phase_voltage_per_switching_state/1 -> Delay32/1
  Delay22/1 -> done/1
  Delay32/1 -> Demux/1
  Data Type Conversion10/1 -> Switch_on13/1
  Data Type Conversion9/1 -> Switch_on15/1
  Data Type Conversion8/1 -> Switch_on16/1
  Data Type Conversion7/1 -> Switch_on17/1
  Data Type Conversion4/1 -> Product/1
  Subsystem/8(J7) -> Data Type Conversion39/1
  Subsystem/7(J6) -> Data Type Conversion40/1
  Subsystem/6(J5) -> Data Type Conversion41/1
  Subsystem/5(J4) -> Data Type Conversion42/1
  Subsystem/4(J3) -> Data Type Conversion43/1
  Subsystem/3(J2) -> Data Type Conversion44/1
  Subsystem/2(J1) -> Data Type Conversion45/1
  Subsystem/1(J) -> Data Type Conversion46/1
  Data Type Conversion38/1 -> Switch_on59/1
  Data Type Conversion37/1 -> Switch_on60/1
  Data Type Conversion36/1 -> Switch_on61/1
  Data Type Conversion35/1 -> Switch_on62/1
  Data Type Conversion34/1 -> Switch_on63/1
  Data Type Conversion33/1 -> Switch_on64/1
  Data Type Conversion32/1 -> Switch_on65/1
  Data Type Conversion31/1 -> Switch_on66/1
  Data Type Conversion30/1 -> Switch_on67/1
  Data Type Conversion29/1 -> Switch_on68/1
  Data Type Conversion28/1 -> Switch_on69/1
  Data Type Conversion27/1 -> Switch_on70/1
  Data Type Conversion26/1 -> Switch_on71/1
  Data Type Conversion25/1 -> Switch_on72/1
  Data Type Conversion24/1 -> Switch_on73/1
  Data Type Conversion23/1 -> Switch_on74/1
  Data Type Conversion22/1 -> Switch_on75/1
  Data Type Conversion21/1 -> Switch_on76/1
  Data Type Conversion20/1 -> Switch_on77/1
  Data Type Conversion19/1 -> Switch_on78/1
  Data Type Conversion17/1 -> Switch_on79/1
  Data Type Conversion16/1 -> Switch_on80/1
  Data Type Conversion15/1 -> Switch_on81/1
  Data Type Conversion14/1 -> Switch_on82/1
  Data Type Conversion13/1 -> Switch_on83/1
  Data Type Conversion12/1 -> Switch_on84/1
  Data Type Conversion11/1 -> Switch_on85/1
  Data Type Conversion6/1 -> Switch_on86/1
  Data Type Conversion5/1 -> Switch_on87/1
  Data Type Conversion3/1 -> Switch_on88/1
  Data Type Conversion2/1 -> Switch_on89/1
  Data Type Conversion1/1 -> Switch_on90/1
  Data Type Conversion39/1 -> Mux/8
  Data Type Conversion40/1 -> Mux/7
  Data Type Conversion41/1 -> Mux/6
  Data Type Conversion42/1 -> Mux/5
  Data Type Conversion43/1 -> Mux/4
  Data Type Conversion44/1 -> Mux/3
  Data Type Conversion45/1 -> Mux/2
  Data Type Conversion46/1 -> Mux/1
  Detect Rise Positive2/1 -> Switch_on4/2, Switch_on11/2  "End_Cycle"
  Switch_on4/1 -> Product/2, Delay4/1
  Delay4/1 -> Switch_on4/3

== system FCS_MPC_6ph_Regelungsmodell/Microcontroller Software/Subsystem2 ==
  i_a1 : Inport
  i_b1 : Inport  Port=2
  i_c1 : Inport  Port=3
  i_a2 : Inport  Port=4
  i_b2 : Inport  Port=5
  i_c2 : Inport  Port=6
  theta_el : Inport  Port=7
  theta_el_offset_AXI : Inport  Port=8
  curent_valid_in : Inport  Port=9
  6ph_PMSM_30deg_VSD1 : MATLAB Function  TreatAsAtomicUnit=on  SystemSampleTime=T_100MHz
  Add1 : Sum  Inputs=+-  OutDataTypeStr=Inherit: Same as accumulator
  Add2 : Sum  Inputs=-+  OutDataTypeStr=Inherit: Same as first input
  Add3 : Sum  OutDataTypeStr=Inherit: Same as first input
  Compare Limit_High : simulink/Logic and Bit Operations/Compare To Constant  relop=>=  const=2*pi  OutDataTypeStr=boolean
  Compare Limit_Low : simulink/Logic and Bit Operations/Compare To Constant  relop=<  const=0  OutDataTypeStr=boolean
  Constant : Constant  Value=2*pi  OutDataTypeStr=fixdt(1,24,20)  SampleTime=T_100MHz
  Constant1 : Constant  Value=2*pi  OutDataTypeStr=fixdt(1,24,20)  SampleTime=T_100MHz
  Data Type Conversion{2..9} (8 alike) : DataTypeConversion  OutDataTypeStr=fixdt(1,18,11)  SaturateOnIntegerOverflow=off  RndMeth=Floor
  Delay{1..6,8} (7 alike) : Delay  DelayLength=1
  Detect Rise Positive : hdlsllib/Logic and Bit Operations/Detect Rise Positive  vinit=0  OutDataTypeStr=boolean
      settings: SourceProductBaseCode=SL
  Switch_Limit_High : Switch  Criteria=u2 > Threshold  OutDataTypeStr=Inherit: Inherit via back propagation  SaturateOnIntegerOverflow=off  InputSameDT=off
  Switch_Limit_Low : Switch  Criteria=u2 > Threshold  OutDataTypeStr=Inherit: Inherit via back propagation  SaturateOnIntegerOverflow=off  InputSameDT=off
  Switch_on{1..6,8} (7 alike) : Switch  Threshold=1  OutDataTypeStr=Inherit: Inherit via back propagation  RndMeth=Simplest  SaturateOnIntegerOverflow=off  InputSameDT=off
  i_alpha : Outport
  i_beta : Outport  Port=2
  i_d : Outport  Port=3
  i_q : Outport  Port=4
  i_x : Outport  Port=5
  i_y : Outport  Port=6
  i_0_plus : Outport  Port=7
  i_0_minus : Outport  Port=8
  done : Outport  Port=9
  wires:
  6ph_PMSM_30deg_VSD1/2(i_beta) -> Data Type Conversion3/1
  6ph_PMSM_30deg_VSD1/7(i_d) -> Data Type Conversion8/1
  6ph_PMSM_30deg_VSD1/1(i_alpha) -> Data Type Conversion2/1
  6ph_PMSM_30deg_VSD1/8(i_q) -> Data Type Conversion9/1
  6ph_PMSM_30deg_VSD1/5(i_0_plus) -> Data Type Conversion6/1
  6ph_PMSM_30deg_VSD1/6(i_0_minus) -> Data Type Conversion7/1
  6ph_PMSM_30deg_VSD1/4(i_y) -> Data Type Conversion5/1
  6ph_PMSM_30deg_VSD1/3(i_x) -> Data Type Conversion4/1
  Delay6/1 -> Switch_on6/3
  Switch_on6/1 -> Delay6/1, 6ph_PMSM_30deg_VSD1/1(i_a1)
  Switch_on1/1 -> Delay1/1, 6ph_PMSM_30deg_VSD1/2(i_b1)
  Delay1/1 -> Switch_on1/3
  Delay2/1 -> Switch_on2/3
  Switch_on2/1 -> Delay2/1, 6ph_PMSM_30deg_VSD1/3(i_c1)
  Delay3/1 -> Switch_on3/3
  Switch_on3/1 -> Delay3/1, 6ph_PMSM_30deg_VSD1/4(i_a2)
  Delay4/1 -> Switch_on4/3
  Switch_on4/1 -> Delay4/1, 6ph_PMSM_30deg_VSD1/5(i_b2)
  Delay5/1 -> Switch_on5/3
  Switch_on5/1 -> Delay5/1, 6ph_PMSM_30deg_VSD1/6(i_c2)
  Detect Rise Positive/1 -> Switch_on6/2, Switch_on1/2, Switch_on2/2, Switch_on3/2, Switch_on4/2, Switch_on5/2, Switch_on8/2, done/1  "End_Cycle"
  Switch_on8/1 -> 6ph_PMSM_30deg_VSD1/7(theta_el), Delay8/1
  Delay8/1 -> Switch_on8/3
  curent_valid_in/1 -> Detect Rise Positive/1  "End_Cycle"
  Switch_Limit_Low/1 -> Switch_on8/1  "End_Cycle"
  Constant1/1 -> Add3/2
  Compare Limit_High/1 -> Switch_Limit_High/2
  Add3/1 -> Switch_Limit_Low/1
  Compare Limit_Low/1 -> Switch_Limit_Low/2
  theta_el_offset_AXI/1 -> Add1/2
  Add1/1 -> Switch_Limit_High/3, Add3/1, Compare Limit_Low/1, Add2/2, Compare Limit_High/1
  Add2/1 -> Switch_Limit_High/1
  Constant/1 -> Add2/1
  Switch_Limit_High/1 -> Switch_Limit_Low/3
  i_a1/1 -> Switch_on6/1  "End_Cycle"
  i_b1/1 -> Switch_on1/1  "End_Cycle"
  i_c1/1 -> Switch_on2/1  "End_Cycle"
  i_a2/1 -> Switch_on3/1  "End_Cycle"
  i_b2/1 -> Switch_on4/1  "End_Cycle"
  i_c2/1 -> Switch_on5/1  "End_Cycle"
  theta_el/1 -> Add1/1  "End_Cycle"
  Data Type Conversion2/1 -> i_alpha/1  "curent_valid_in"
  Data Type Conversion3/1 -> i_beta/1  "curent_valid_in"
  Data Type Conversion4/1 -> i_x/1  "curent_valid_in"
  Data Type Conversion5/1 -> i_y/1  "curent_valid_in"
  Data Type Conversion6/1 -> i_0_plus/1  "curent_valid_in"
  Data Type Conversion7/1 -> i_0_minus/1  "curent_valid_in"
  Data Type Conversion8/1 -> i_d/1  "curent_valid_in"
  Data Type Conversion9/1 -> i_q/1  "curent_valid_in"

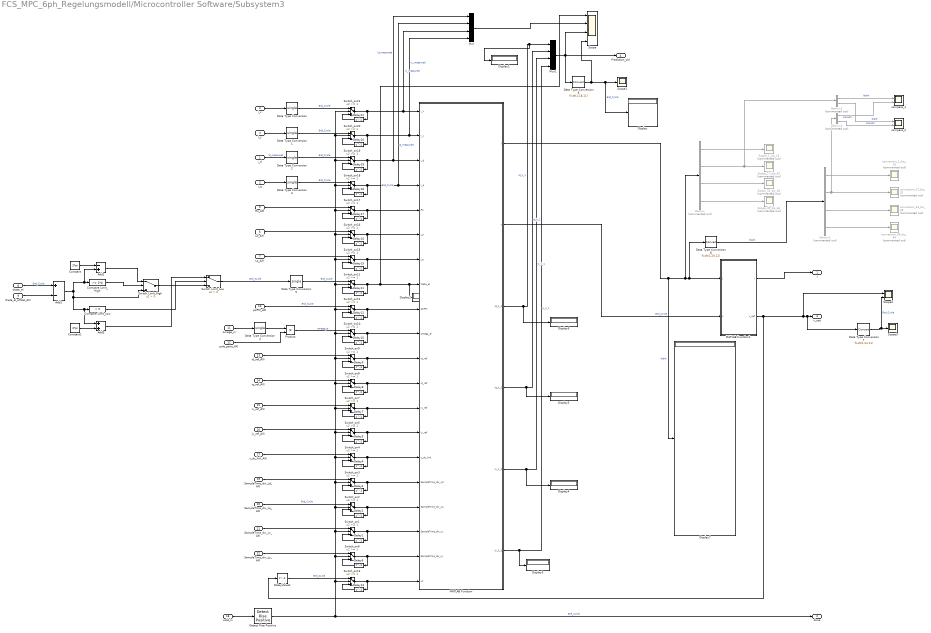
== system FCS_MPC_6ph_Regelungsmodell/Microcontroller Software/Subsystem3 ==
  i_d : Inport
  i_q : Inport  Port=2
  i_x : Inport  Port=3
  i_y : Inport  Port=4
  Rs_AXI : Inport  Port=5
  Ld_AXI : Inport  Port=6
  Lq_AXI : Inport  Port=7
  theta_el : Inport  Port=8
  theta_el_offset_AXI : Inport  Port=9
  psiPM_AXI : Inport  Port=10
  omega_m : Inport  Port=11
  pole_pairs_AXI : Inport  Port=12
  id_ref_AXI : Inport  Port=13
  iq_ref_AXI : Inport  Port=14
  ix_ref_AXI : Inport  Port=15
  iy_ref_AXI : Inport  Port=16
  u_dc_link_AXI : Inport  Port=17
  valid_in : Inport  Port=18
  SampleTime_div_Ld_AXI : Inport  Port=19
  SampleTime_div_Lq_AXI : Inport  Port=20
  SampleTime_div_Lx_AXI : Inport  Port=21
  SampleTime_div_Ly_AXI : Inport  Port=22
  Add1 : Sum  Inputs=+-  OutDataTypeStr=Inherit: Same as accumulator
  Add2 : Sum  Inputs=-+  OutDataTypeStr=Inherit: Same as first input
  Add3 : Sum  OutDataTypeStr=Inherit: Same as first input
  Compare Limit_High : simulink/Logic and Bit Operations/Compare To Constant  relop=>=  const=2*pi  OutDataTypeStr=boolean
  Compare Limit_Low : simulink/Logic and Bit Operations/Compare To Constant  relop=<  const=0  OutDataTypeStr=boolean
  Constant : Constant  Value=2*pi  OutDataTypeStr=single  SampleTime=T_100MHz
  Constant1 : Constant  Value=2*pi  OutDataTypeStr=single  SampleTime=T_100MHz
  Data Type Conversion{,1..5} (6 alike) : DataTypeConversion  OutDataTypeStr=single  RndMeth=Nearest  SaturateOnIntegerOverflow=off
  Data Type Conversion6 : DataTypeConversion  OutDataTypeStr=fixdt(1,18,11)  RndMeth=Nearest  SaturateOnIntegerOverflow=off
  Data Type Conversion7 : DataTypeConversion  OutDataTypeStr=fixdt(1,24,11)  RndMeth=Nearest  SaturateOnIntegerOverflow=off
  Data Type Conversion8 : DataTypeConversion  OutDataTypeStr=fixdt(1,20,11)  RndMeth=Nearest  SaturateOnIntegerOverflow=off
  Delay{1..13,15..21} (20 alike) : Delay  DelayLength=1
  DelayValue1 : Delay  DelayLength=1
  Demux : Demux  Commented=on
  Demux1 : Demux  Commented=on
  Demux2 : Demux  Commented=on  Outputs=2
  Demux3 : Demux  Commented=on  Outputs=2
  Detect Rise Positive : hdlsllib/Logic and Bit Operations/Detect Rise Positive  vinit=0  OutDataTypeStr=boolean
      settings: SourceProductBaseCode=SL
  Display{,1..7} (8 alike) : Display
  MATLAB Function : MATLAB Function  TreatAsAtomicUnit=on  SystemSampleTime=T_100MHz
  MATLAB Function1 : MATLAB Function  TreatAsAtomicUnit=on  SystemSampleTime=T_100MHz
  Mux : Mux
  Mux1 : Mux
  Product : Product  Inputs=**
  Scope : Scope  NumInputPorts=4
  Scope1 : Scope
  Scope2 : Scope  NumInputPorts=2
  Scope3 : Scope
  Scope_17_bis_32 : Scope  Commented=on
  Scope_1_bis_16 : Scope  Commented=on
  Scope_33_bis_48 : Scope  Commented=on
  Scope_49_bis_64 : Scope  Commented=on
  Switch_Limit_High : Switch  Criteria=u2 > Threshold  OutDataTypeStr=single  SaturateOnIntegerOverflow=off  InputSameDT=off
  Switch_Limit_Low : Switch  Criteria=u2 > Threshold  OutDataTypeStr=single  SaturateOnIntegerOverflow=off  InputSameDT=off
  Switch_on{1..13,15..21} (20 alike) : Switch  Threshold=1  OutDataTypeStr=single  RndMeth=Simplest  SaturateOnIntegerOverflow=off  InputSameDT=off
  compare_1 : Scope  NumInputPorts=2
  compare_2 : Scope  NumInputPorts=2
  conversion_17_bis_32 : Scope  Commented=on
  conversion_1_bis_16 : Scope  Commented=on
  conversion_33_bis_48 : Scope  Commented=on
  conversion_49_bis_64 : Scope  Commented=on
  I : Outport
  done : Outport  Port=2
  v_opt : Outport  Port=3
  Prediction_old : Outport  Port=4
  wires:
  Product/1 -> Switch_on10/1  "omega_el"
  MATLAB Function/2(v) -> MATLAB Function1/2(v)  "End_Cycle"
  i_d/1 -> Data Type Conversion2/1  "id_measured"
  omega_m/1 -> Data Type Conversion4/1
  i_y/1 -> Data Type Conversion1/1
  i_q/1 -> Data Type Conversion3/1
  i_x/1 -> Data Type Conversion/1
  MATLAB Function1/1(I) -> I/1
  MATLAB Function/1(J) -> Display7/1, Demux/1, MATLAB Function1/1(J), Data Type Conversion8/1  "blank"
  pole_pairs_AXI/1 -> Product/2
  Data Type Conversion4/1 -> Product/1
  valid_in/1 -> Detect Rise Positive/1
  Delay6/1 -> Switch_on6/3
  SampleTime_div_Ly_AXI/1 -> Switch_on6/1
  Switch_on6/1 -> Delay6/1, MATLAB Function/19(SampleTime_div_Ly)
  MATLAB Function1/2(v_opt) -> DelayValue1/1, Scope2/1, Data Type Conversion7/1, v_opt/1
  SampleTime_div_Lx_AXI/1 -> Switch_on1/1
  Delay1/1 -> Switch_on1/3
  Switch_on1/1 -> MATLAB Function/18(SampleTime_div_Lx), Delay1/1
  Delay2/1 -> Switch_on2/3
  Switch_on2/1 -> Delay2/1, MATLAB Function/17(SampleTime_div_Lq)
  SampleTime_div_Ld_AXI/1 -> Switch_on3/1
  Delay3/1 -> Switch_on3/3
  Switch_on3/1 -> MATLAB Function/16(SampleTime_div_Ld), Delay3/1
  u_dc_link_AXI/1 -> Switch_on4/1
  Delay4/1 -> Switch_on4/3
  Switch_on4/1 -> Delay4/1, MATLAB Function/15(u_dc_link)
  iy_ref_AXI/1 -> Switch_on5/1
  SampleTime_div_Lq_AXI/1 -> Switch_on2/1  "End_Cycle"
  Delay5/1 -> Switch_on5/3
  Switch_on5/1 -> MATLAB Function/14(iy_ref), Delay5/1
  ix_ref_AXI/1 -> Switch_on7/1
  Delay7/1 -> Switch_on7/3
  Switch_on7/1 -> MATLAB Function/13(ix_ref), Delay7/1
  iq_ref_AXI/1 -> Switch_on8/1
  Delay8/1 -> Switch_on8/3
  Switch_on8/1 -> MATLAB Function/12(iq_ref), Delay8/1
  id_ref_AXI/1 -> Switch_on9/1
  Delay9/1 -> Switch_on9/3
  Switch_on9/1 -> MATLAB Function/11(id_ref), Delay9/1
  Delay10/1 -> Switch_on10/3
  Switch_on10/1 -> Delay10/1, MATLAB Function/10(omega_el)
  Delay12/1 -> Switch_on12/3
  Switch_on12/1 -> MATLAB Function/9(psiPM), Delay12/1
  psiPM_AXI/1 -> Switch_on12/1  "End_Cycle"
  Lq_AXI/1 -> Switch_on15/1
  Delay15/1 -> Switch_on15/3
  Switch_on15/1 -> Delay15/1, MATLAB Function/7(Lq)
  Ld_AXI/1 -> Switch_on16/1
  Delay16/1 -> Switch_on16/3
  Switch_on16/1 -> MATLAB Function/6(Ld), Delay16/1
  Rs_AXI/1 -> Switch_on17/1
  Delay17/1 -> Switch_on17/3
  Switch_on17/1 -> Delay17/1, MATLAB Function/5(Rs)
  Delay18/1 -> Switch_on18/3
  Switch_on18/1 -> MATLAB Function/4(i_q), Mux/2, Delay18/1  "iq_measured"
  Delay19/1 -> Switch_on19/3
  Switch_on19/1 -> Mux/1, MATLAB Function/3(i_d), Delay19/1  "id_measured"
  Delay20/1 -> Switch_on20/3
  Switch_on20/1 -> Delay20/1, MATLAB Function/2(i_y), Mux/4  "iy_measured"
  Delay21/1 -> Switch_on21/3
  Switch_on21/1 -> Delay21/1, MATLAB Function/1(i_x), Mux/3  "ix_measured"
  Delay11/1 -> Switch_on11/3
  Data Type Conversion5/1 -> Switch_on11/1  "End_Cycle"
  DelayValue1/1 -> Switch_on13/1  "End_Cycle"
  Detect Rise Positive/1 -> Switch_on13/2, Switch_on3/2, Switch_on4/2, Switch_on21/2, Switch_on20/2, Switch_on19/2, Switch_on18/2, Switch_on17/2, Switch_on16/2, Switch_on15/2, Switch_on11/2, Switch_on12/2, Switch_on10/2, Switch_on9/2, Switch_on8/2, Switch_on7/2, Switch_on5/2, Switch_on2/2, Switch_on1/2, Switch_on6/2, done/1  "End_Cycle"
  Delay13/1 -> Switch_on13/3
  Switch_on13/1 -> MATLAB Function/20(vk), Delay13/1
  MATLAB Function/3(id_k_1) -> Display6/1, Display1/1, Mux1/1  "id_k_1"
  MATLAB Function/4(iq_k_1) -> Display5/1, Mux1/2  "iq_k_1"
  MATLAB Function/5(ix_k_1) -> Display4/1, Mux1/3  "ix_k_1"
  MATLAB Function/6(iy_k_1) -> Display3/1, Mux1/4  "iy_k_1"
  Mux1/1 -> Prediction_old/1, Data Type Conversion6/1, Scope/3
  Mux/1 -> Scope/2
  Data Type Conversion/1 -> Switch_on21/1  "End_Cycle"
  Data Type Conversion1/1 -> Switch_on20/1  "End_Cycle"
  Data Type Conversion2/1 -> Switch_on19/1  "End_Cycle"
  Data Type Conversion3/1 -> Switch_on18/1  "End_Cycle"
  Switch_on11/1 -> Scope/1, Display2/1, MATLAB Function/8(theta_el), Delay11/1  "End_Cycle"
  Switch_Limit_Low/1 -> Data Type Conversion5/1  "End_Cycle"
  theta_el_offset_AXI/1 -> Add1/2
  Switch_Limit_High/1 -> Switch_Limit_Low/3
  Add1/1 -> Switch_Limit_High/3, Add3/1, Compare Limit_Low/1, Add2/2, Compare Limit_High/1
  Add2/1 -> Switch_Limit_High/1
  Compare Limit_Low/1 -> Switch_Limit_Low/2
  Compare Limit_High/1 -> Switch_Limit_High/2
  Add3/1 -> Switch_Limit_Low/1
  Constant/1 -> Add2/1
  Constant1/1 -> Add3/2
  theta_el/1 -> Add1/1  "End_Cycle"
  Data Type Conversion6/1 -> Scope/4, Display/1, Scope1/1  "End_Cycle"
  Data Type Conversion7/1 -> Scope2/2, Scope3/1  "End_Cycle"
  Demux/1 -> Scope_1_bis_16/1
  Demux/2 -> Demux2/1, Scope_17_bis_32/1
  Demux/3 -> Scope_33_bis_48/1
  Demux/4 -> Scope_49_bis_64/1
  Demux1/4 -> conversion_49_bis_64/1
  Demux1/3 -> conversion_33_bis_48/1
  Demux1/1 -> conversion_1_bis_16/1
  Demux1/2 -> conversion_17_bis_32/1, Demux3/1
  Data Type Conversion8/1 -> Demux1/1  "blank"
  Demux2/1 -> compare_1/1  "blank"
  Demux3/1 -> compare_1/2  "convert"
  Demux2/2 -> compare_2/1  "blank"
  Demux3/2 -> compare_2/2  "convert"

== system FCS_MPC_6ph_Regelungsmodell/Microcontroller Software/Subsystem5 ==
  I : Inport
  valid_in : Inport  Port=2
  Delay2 : Delay  DelayLength=1
  Demux : Demux  Outputs=12
  Detect Rise Positive : hdlsllib/Logic and Bit Operations/Detect Rise Positive  vinit=0  OutDataTypeStr=boolean
      settings: SourceProductBaseCode=SL
  MATLAB Function1 : MATLAB Function  TreatAsAtomicUnit=on
  Switch_on2 : Switch  Threshold=1  OutDataTypeStr=Inherit: Inherit via back propagation  RndMeth=Simplest  SaturateOnIntegerOverflow=off  InputSameDT=off
  HB1T : Outport
  HB1B : Outport  Port=2
  HB2T : Outport  Port=3
  HB2B : Outport  Port=4
  HB3T : Outport  Port=5
  HB3B : Outport  Port=6
  HB4T : Outport  Port=7
  HB4B : Outport  Port=8
  HB5T : Outport  Port=9
  HB5B : Outport  Port=10
  HB6T : Outport  Port=11
  HB6B : Outport  Port=12
  done : Outport  Port=13
  wires:
  MATLAB Function1/1(next_switching_state) -> Demux/1
  Switch_on2/1 -> MATLAB Function1/1(I), Delay2/1
  Delay2/1 -> Switch_on2/3
  I/1 -> Switch_on2/1
  valid_in/1 -> Detect Rise Positive/1
  Detect Rise Positive/1 -> done/1, Switch_on2/2  "End_Cycle"
  Demux/1 -> HB1T/1
  Demux/2 -> HB1B/1
  Demux/3 -> HB2T/1
  Demux/4 -> HB2B/1
  Demux/5 -> HB3T/1
  Demux/6 -> HB3B/1
  Demux/7 -> HB4T/1
  Demux/8 -> HB4B/1
  Demux/9 -> HB5T/1
  Demux/10 -> HB5B/1
  Demux/11 -> HB6T/1
  Demux/12 -> HB6B/1
